simulink model "COR_test"  (Simulink 7.4)
settings: Solver=FixedStepDiscrete  StartTime=0.0  StopTime=1e6  FixedStep=0.01  RelTol=1e-3
libraries: COR_lib x1, simulink x1
settings Model: Creator=Administrator  LastModifiedBy=sunsijun
settings DataIOCC: SaveFormat=Structure
settings OptimizationCC: InitFltsAndDblsToZero=on
settings DebuggingCC: InheritedTsInSrcMsg=none  ParameterPrecisionLossMsg=none
settings RTWCC: GenCodeOnly=on

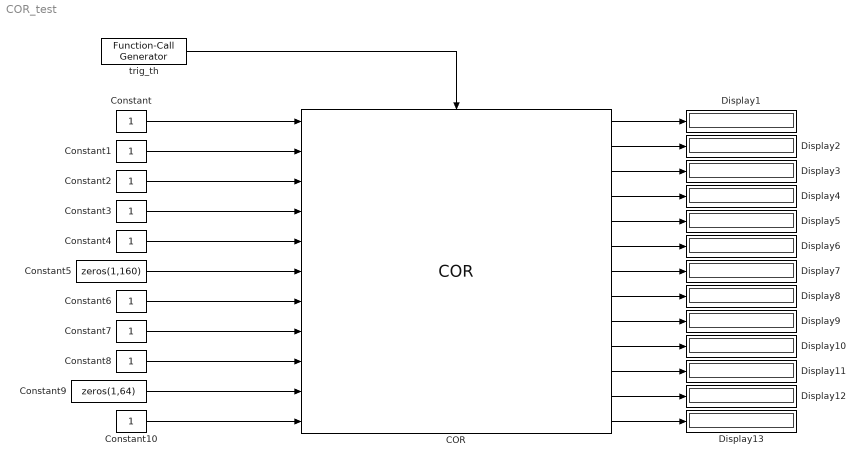
== system COR_test ==
  COR : COR_lib/COR  SystemSampleTime=-1
  Constant : Constant  OutDataTypeMode=uint8  OutDataType=fixdt(1, 16)  OutScaling=2^0  OutDataTypeStr=uint8
  Constant{1..3,6..7,10} (6 alike) : Constant  OutDataTypeMode=single  OutDataType=fixdt(1, 16)  OutScaling=2^0  OutDataTypeStr=single
  Constant4 : Constant  OutDataTypeMode=uint16  OutDataType=fixdt(1, 16)  OutScaling=2^0  OutDataTypeStr=uint16
  Constant5 : Constant  Value=zeros(1,160)  OutDataTypeMode=single  OutDataType=fixdt(1, 16)  OutScaling=2^0  OutDataTypeStr=single
  Constant8 : Constant  OutDataTypeMode=boolean  OutDataType=fixdt(1, 16)  OutScaling=2^0  OutDataTypeStr=boolean
  Constant9 : Constant  Value=zeros(1,64)  OutDataTypeMode=single  OutDataType=fixdt(1, 16)  OutScaling=2^0  OutDataTypeStr=single
  Display{1..13} (13 alike) : Display
  trig_th : simulink/Ports & Subsystems/Function-Call Generator  sample_time=-1  numberOfIterations=1
  wires:
  trig_th/1 -> COR/Trigger
  Constant/1 -> COR/1
  Constant1/1 -> COR/2
  Constant2/1 -> COR/3
  Constant3/1 -> COR/4
  Constant4/1 -> COR/5
  Constant5/1 -> COR/6
  Constant6/1 -> COR/7
  Constant7/1 -> COR/8
  Constant8/1 -> COR/9
  Constant9/1 -> COR/10
  Constant10/1 -> COR/11
  COR/1 -> Display1/1
  COR/2 -> Display2/1
  COR/3 -> Display3/1
  COR/4 -> Display4/1
  COR/5 -> Display5/1
  COR/6 -> Display6/1
  COR/7 -> Display7/1
  COR/8 -> Display8/1
  COR/9 -> Display9/1
  COR/10 -> Display10/1
  COR/11 -> Display11/1
  COR/12 -> Display12/1
  COR/13 -> Display13/1
